simulink model "SimulateurNL_Pont_Cmd_LQ"  (R2022b)
settings: Solver=VariableStepAuto  StartTime=0.0  StopTime=30  MaxStep=0.001  RelTol=1e-3
values from neighbouring files (symbols this model uses):
  a = [0.488]    [Validation_param_pend.m]    (also in code.m = 0.0487)
  f = 7.25e-5    (= 7.25e-05)    [code.m]
  g = 9.81    [code.m]
  J = 3.9e-6    (= 3.9e-06)    [code.m]
  K_lq = lqr(Ap,Bp,Q_lq,R_lq)    [code.m]
  Kfi = 4.77    [code.m]
  Ki = 5    [code.m]
  Komga = 0.02    [code.m]
  Kteta = 0.875    [code.m]
  Kv = [43]    [Validation_KvTaum.m]    (also in code.m = 43.3)
  l = [0.2687]    [Validation_param_pend.m]    (also in code.m = 0.2687)
  Lm = 0.2e-3    (= 0.0002)    [code.m]
  M_lq = -inv(Cp(1,:)*inv(Ap-Bp*K_lq)*Bp)    [code.m]
  N = 17    [Validation_param_pend.m]    (also in code.m)
  r = 0.022    [Validation_param_pend.m]    (also in code.m)
  Rm = 2.25    [code.m]
  Taum = [0.035]    [Validation_KvTaum.m]    (also in code.m = 0.035)
  Te1 = 0.100    (= 0.1)    [code.m]    (also in matlab.mat = 0)
libraries: simulink_extras x1
settings Model: Creator=Godoy  LastModifiedBy=Pedro
settings SolverCC: AlgebraicLoopSolver=TrustRegion
settings DataIOCC: ReturnWorkspaceOutputs=off
settings DebuggingCC: UnconnectedInputMsg=warning  UnconnectedOutputMsg=warning  UnconnectedLineMsg=warning  SFMachineParentedDataDiag=warning  ArithmeticOperatorsInVariantConditions=warning
settings ModelReferenceCC: EnableRefExpFcnMdlSchedulingChecks=on
settings SFSimCC: CustomCodeUndefinedFunction=UseInterfaceOnly

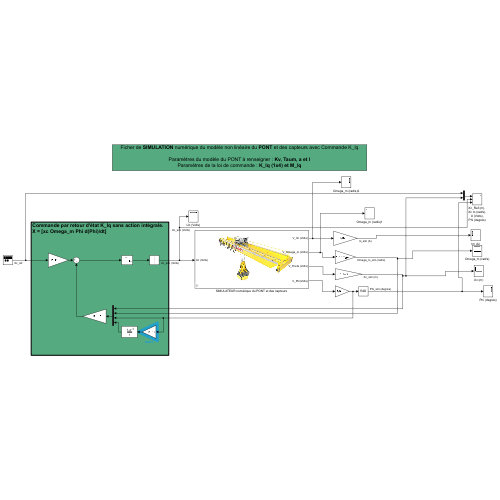
[thumbnail: Simulink's stored preview of the top-level diagram]
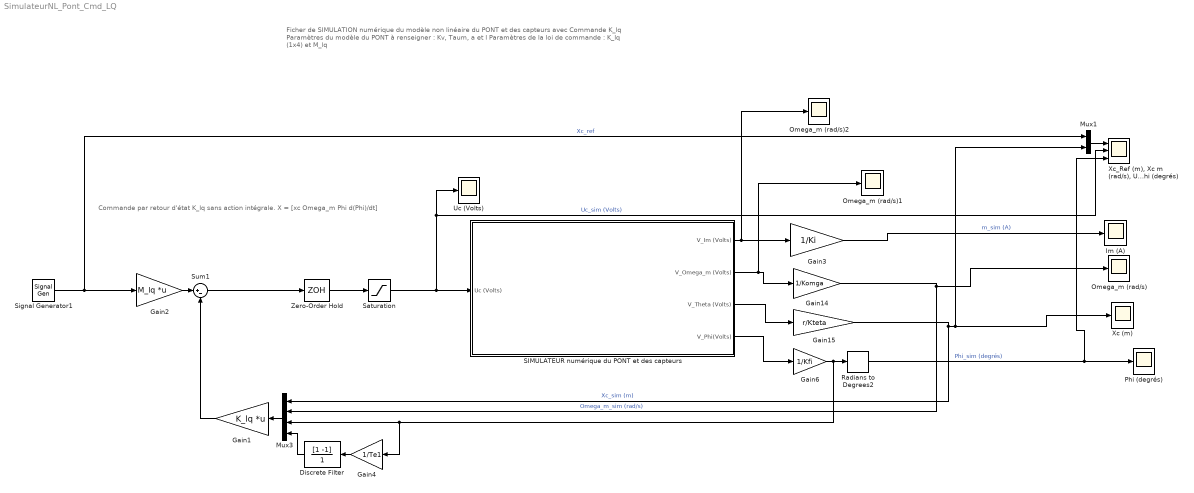
== system SimulateurNL_Pont_Cmd_LQ ==
  note: Commande par retour d'état K_lq sans action intégrale.
      | X = [xc Omega_m Phi d(Phi)/dt]
  note: Ficher de SIMULATION numérique du modèle non linéaire du PONT et des capteurs avec Commande K_lq
      |
      | Paramètres du modèle du PONT à renseigner : Kv, Taum, a et l
      | Paramètres de la loi de commande : K_lq (1x4) et M_lq
  Discrete Filter : DiscreteFilter  Numerator=[1 -1]  Denominator=1  SampleTime=Te1
  Gain1 : Gain  Gain=K_lq  Multiplication=Matrix(K*u)
  Gain14 : Gain  Gain=1/Komga
  Gain15 : Gain  Gain=r/Kteta
  Gain2 : Gain  Gain=M_lq  Multiplication=Matrix(K*u)
  Gain3 : Gain  Gain=1/Ki
  Gain4 : Gain  Gain=1/Te1
  Gain6 : Gain  Gain=1/Kfi
  Im (A) : Scope
  Mux1 : Mux  Inputs=2
  Mux3 : Mux
  Omega_m (rad/s) : Scope
  Omega_m (rad/s)1 : Scope
  Omega_m (rad/s)2 : Scope
  Phi (degrés) : Scope
  Radians to Degrees2 : simulink_extras/Transformations/Radians to Degrees
  "SIMULATEUR numérique du PONT et des capteurs " : Subsystem  mask{Kv=Kv, Taum=Taum, a=a, l=l}
      mask prompts: l "longueur l (m)"
      mask Display: image('$imagefile'); % Use "Edit Image" on toolstrip to change.
  Saturation : Saturate  UpperLimit=9.99  LowerLimit=-9.99
  Signal Generator1 : SignalGenerator  WaveForm=square  Amplitude=0.15  Frequency=0.1
  Sum1 : Sum  Inputs=|+-
  Uc (Volts) : Scope
  Xc (m) : Scope
  "Xc_Ref (m), Xc m (rad/s), U (Volts), Phi (degrés)" : Scope  NumInputPorts=3
  Zero-Order Hold : ZeroOrderHold  SampleTime=Te1
  wires:
  Gain14/1 -> Mux3/2, Omega_m (rad/s)/1  "Omega_m_sim (rad/s)"
  "SIMULATEUR numérique du PONT et des capteurs "/3(V_Theta (Volts)) -> Gain15/1
  "SIMULATEUR numérique du PONT et des capteurs "/4(V_Phi(Volts)) -> Gain6/1
  "SIMULATEUR numérique du PONT et des capteurs "/2(V_Omega_m (Volts)) -> Omega_m (rad/s)1/1, Gain14/1
  Radians to Degrees2/1 -> "Xc_Ref (m), Xc m (rad/s), U (Volts), Phi (degrés)"/3, Phi (degrés)/1  "Phi_sim (degrés)"
  "SIMULATEUR numérique du PONT et des capteurs "/1(V_Im (Volts)) -> Omega_m (rad/s)2/1, Gain3/1
  Gain6/1 -> Gain4/1, Mux3/3, Radians to Degrees2/1
  Gain3/1 -> Im (A)/1  "m_sim (A)"
  Saturation/1 -> "SIMULATEUR numérique du PONT et des capteurs "/1(Uc (Volts)), "Xc_Ref (m), Xc m (rad/s), U (Volts), Phi (degrés)"/2, Uc (Volts)/1  "Uc_sim (Volts)"
  Zero-Order Hold/1 -> Saturation/1
  Gain1/1 -> Sum1/2
  Gain15/1 -> Mux3/1, Mux1/2, Xc (m)/1  "Xc_sim (m)"
  Mux3/1 -> Gain1/1
  Gain2/1 -> Sum1/1
  Signal Generator1/1 -> Mux1/1, Gain2/1  "Xc_ref"
  Mux1/1 -> "Xc_Ref (m), Xc m (rad/s), U (Volts), Phi (degrés)"/1
  Sum1/1 -> Zero-Order Hold/1
  Discrete Filter/1 -> Mux3/4
  Gain4/1 -> Discrete Filter/1

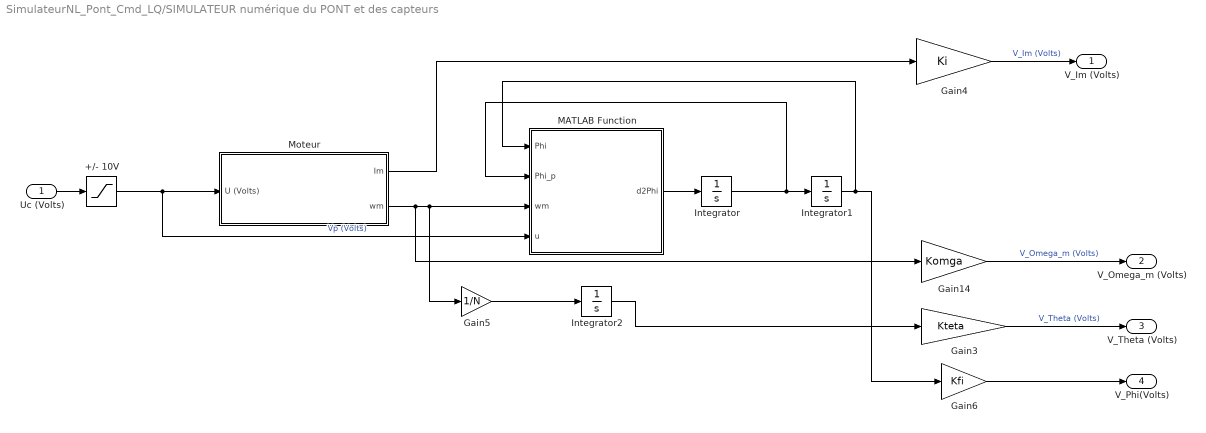
== system SimulateurNL_Pont_Cmd_LQ/SIMULATEUR numérique du PONT et des capteurs  ==
  Uc (Volts) : Inport
  +/- 10V : Saturate  UpperLimit=10  LowerLimit=-10
  Gain14 : Gain  Gain=Komga
  Gain3 : Gain  Gain=Kteta
  Gain4 : Gain  Gain=Ki
  Gain5 : Gain  Gain=1/N
  Gain6 : Gain  Gain=Kfi
  Integrator : Integrator
  Integrator1 : Integrator
  Integrator2 : Integrator
  MATLAB Function : MATLAB Function  TreatAsAtomicUnit=on
  Moteur : Subsystem
  V_Im (Volts) : Outport
  V_Omega_m (Volts) : Outport  Port=2
  V_Theta (Volts) : Outport  Port=3
  V_Phi(Volts) : Outport  Port=4
  wires:
  Uc (Volts)/1 -> +/- 10V/1
  Gain14/1 -> V_Omega_m (Volts)/1  "V_Omega_m (Volts)"
  Moteur/2(wm) -> Gain14/1, Gain5/1, MATLAB Function/3(wm)
  Gain5/1 -> Integrator2/1
  MATLAB Function/1(d2Phi) -> Integrator/1
  Moteur/1(Im) -> Gain4/1
  Integrator/1 -> MATLAB Function/2(Phi_p), Integrator1/1
  Integrator1/1 -> Gain6/1, MATLAB Function/1(Phi)
  Gain6/1 -> V_Phi(Volts)/1
  Integrator2/1 -> Gain3/1
  Gain4/1 -> V_Im (Volts)/1  "V_Im (Volts)"
  Gain3/1 -> V_Theta (Volts)/1  "V_Theta (Volts)"
  +/- 10V/1 -> MATLAB Function/4(u), Moteur/1(U (Volts))  "Vp (Volts)"

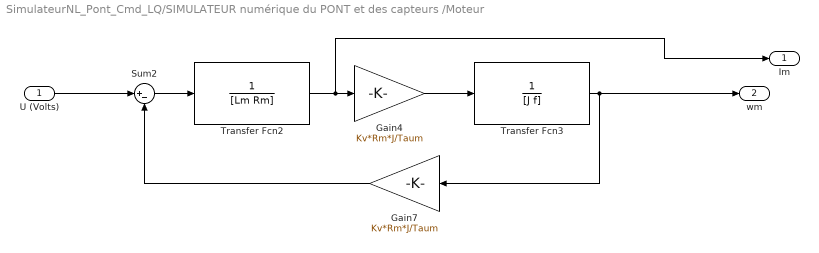
== system SimulateurNL_Pont_Cmd_LQ/SIMULATEUR numérique du PONT et des capteurs /Moteur ==
  U (Volts) : Inport
  Gain4 : Gain  Gain=Kv*Rm*J/Taum
  Gain7 : Gain  Gain=Kv*Rm*J/Taum
  Sum2 : Sum  Inputs=|+-
  Transfer Fcn2 : TransferFcn  Denominator=[Lm Rm]
  Transfer Fcn3 : TransferFcn  Denominator=[J f]
  Im : Outport
  wm : Outport  Port=2
  wires:
  U (Volts)/1 -> Sum2/1
  Gain7/1 -> Sum2/2
  Transfer Fcn2/1 -> Gain4/1, Im/1
  Sum2/1 -> Transfer Fcn2/1
  Gain4/1 -> Transfer Fcn3/1
  Transfer Fcn3/1 -> Gain7/1, wm/1

== matlab function SimulateurNL_Pont_Cmd_LQ/SIMULATEUR numérique du PONT et des capteurs /MATLAB Function ==
  data: Phi input; Phi_p input; wm input; u input; d2Phi output size=1; r parameter; N parameter; l parameter; a parameter; Taum parameter; Kv parameter; g parameter
function d2Phi = fcn(Phi, Phi_p, wm, u, r, N, l, a, Taum, Kv, g)

d2Phi=(-r/N*cos(Phi)*(-1/Taum*wm+Kv/Taum*u)-g*sin(Phi) -a*Phi_p)/l;
